simulink model "GradingSystem"  (R2021a)
settings: Solver=FixedStepDiscrete  StartTime=0.0  StopTime=10.0  RelTol=1e-3  EnableMultiTasking=on
settings Model: Creator=Karim  LastModifiedBy=Karim
settings DataIOCC: ReturnWorkspaceOutputs=off
settings OptimizationCC: DefaultParameterBehavior=Inlined  InlineInvariantSignals=on  EnableMemcpy=off  LifeSpan=1  EfficientTunableParamExpr=on
settings DebuggingCC: UnderspecifiedInitializationDetection=Classic  MergeDetectMultiDrivingBlocksExec=none  SFMachineParentedDataDiag=warning  ArithmeticOperatorsInVariantConditions=warning
settings ModelReferenceCC: PropagateSignalLabelsOutOfModel=off
settings SFSimCC: MATLABDynamicMemAlloc=off  CustomCodeUndefinedFunction=UseInterfaceOnly
settings RTWCC: SystemTargetFile=ert.tlc  GenCodeOnly=on  TemplateMakefile=ert_default_tmf  GenerateReport=on  IncludeHyperlinkInReport=on  LaunchReport=on  GenerateTraceInfo=on  GenerateTraceReport=on  GenerateTraceReportSl=on  GenerateTraceReportSf=on  GenerateTraceReportEml=on
settings CodeAppCC: ForceParamTrailComments=on  IgnoreCustomStorageClasses=off  OperatorAnnotations=on  SimulinkDataObjDesc=on  SFDataObjDesc=on  MATLABFcnDesc=on  InsertBlockDesc=on  StateflowObjectComments=on  MATLABSourceComments=on
settings ERTTargetCC: MultiwordLength=2048  GenerateSampleERTMain=on  InlinedParameterPlacement=NonHierarchical  ERTCustomFileTemplate=example_file_process.tlc

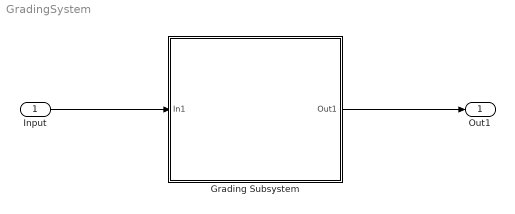
== system GradingSystem ==
  Input : Inport  OutMax=100  OutDataTypeStr=int8
  Grading Subsystem : Subsystem
  Out1 : Outport
  wires:
  Grading Subsystem/1(Out1) -> Out1/1
  Input/1 -> Grading Subsystem/1(In1)

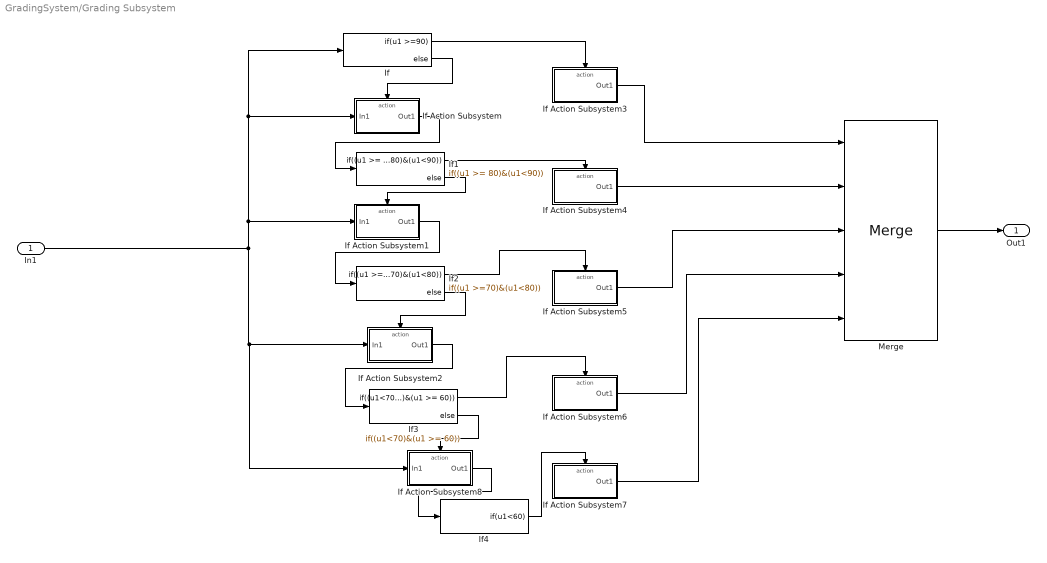
== system GradingSystem/Grading Subsystem ==
  In1 : Inport
  If : If  IfExpression=u1 >=90
  If Action Subsystem : Subsystem  TreatAsAtomicUnit=on
  If Action Subsystem1 : Subsystem  TreatAsAtomicUnit=on
  If Action Subsystem2 : Subsystem  TreatAsAtomicUnit=on
  If Action Subsystem3 : Subsystem  TreatAsAtomicUnit=on
  If Action Subsystem4 : Subsystem  TreatAsAtomicUnit=on
  If Action Subsystem5 : Subsystem  TreatAsAtomicUnit=on
  If Action Subsystem6 : Subsystem  TreatAsAtomicUnit=on
  If Action Subsystem7 : Subsystem  TreatAsAtomicUnit=on
  If Action Subsystem8 : Subsystem  TreatAsAtomicUnit=on
  If1 : If  IfExpression=(u1 >= 80)&(u1<90)
  If2 : If  IfExpression=(u1 >=70)&(u1<80)
  If3 : If  IfExpression=(u1<70)&(u1 >= 60)
  If4 : If  IfExpression=u1<60  ShowElse=off
  Merge : Merge  Inputs=5
  Out1 : Outport
  wires:
  If/2 -> If Action Subsystem/Action
  If Action Subsystem3/1(Out1) -> Merge/1
  If4/1 -> If Action Subsystem7/Action
  If Action Subsystem8/1(Out1) -> If4/1
  If Action Subsystem7/1(Out1) -> Merge/5
  If Action Subsystem5/1(Out1) -> Merge/3
  In1/1 -> If/1, If Action Subsystem/1(In1), If Action Subsystem1/1(In1), If Action Subsystem8/1(In1), If Action Subsystem2/1(In1)
  If Action Subsystem4/1(Out1) -> Merge/2
  If Action Subsystem/1(Out1) -> If1/1
  If Action Subsystem2/1(Out1) -> If3/1
  If Action Subsystem6/1(Out1) -> Merge/4
  If3/2 -> If Action Subsystem8/Action
  If1/2 -> If Action Subsystem1/Action
  If3/1 -> If Action Subsystem6/Action
  If/1 -> If Action Subsystem3/Action
  If2/1 -> If Action Subsystem5/Action
  If Action Subsystem1/1(Out1) -> If2/1
  If2/2 -> If Action Subsystem2/Action
  If1/1 -> If Action Subsystem4/Action
  Merge/1 -> Out1/1

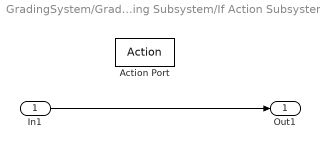
== system GradingSystem/Grading Subsystem/If Action Subsystem ==
  In1 : Inport
  Action Port : ActionPort  ActionPortLabel=else
  Out1 : Outport
  wires:
  In1/1 -> Out1/1

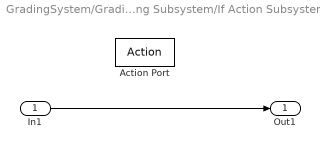
== system GradingSystem/Grading Subsystem/If Action Subsystem1 ==
  In1 : Inport
  Action Port : ActionPort  ActionPortLabel=else
  Out1 : Outport
  wires:
  In1/1 -> Out1/1

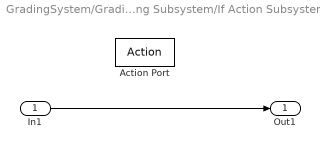
== system GradingSystem/Grading Subsystem/If Action Subsystem2 ==
  In1 : Inport
  Action Port : ActionPort  ActionPortLabel=else
  Out1 : Outport
  wires:
  In1/1 -> Out1/1

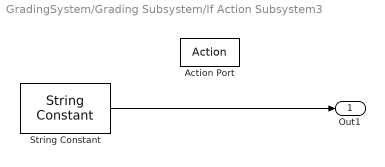
== system GradingSystem/Grading Subsystem/If Action Subsystem3 ==
  Action Port : ActionPort  ActionPortLabel=if(u1 >=90)
  String Constant : StringConstant  String="\"A\""
  Out1 : Outport
  wires:
  String Constant/1 -> Out1/1

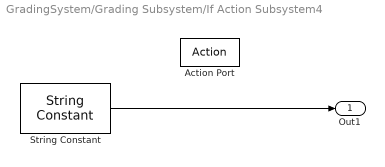
== system GradingSystem/Grading Subsystem/If Action Subsystem4 ==
  Action Port : ActionPort  ActionPortLabel=if((u1 >= 80)&(u1<90))
  String Constant : StringConstant  String="\"B\""
  Out1 : Outport
  wires:
  String Constant/1 -> Out1/1

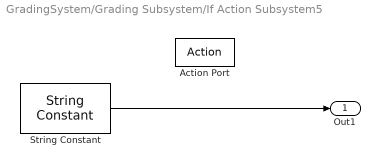
== system GradingSystem/Grading Subsystem/If Action Subsystem5 ==
  Action Port : ActionPort  ActionPortLabel=if((u1 >=70)&(u1<80))
  String Constant : StringConstant  String="\"C\""
  Out1 : Outport
  wires:
  String Constant/1 -> Out1/1

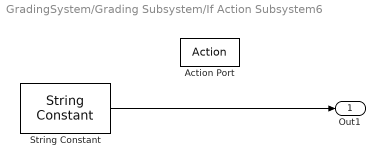
== system GradingSystem/Grading Subsystem/If Action Subsystem6 ==
  Action Port : ActionPort  ActionPortLabel=if((u1<70)&(u1 >= 60))
  String Constant : StringConstant  String="\"D\""
  Out1 : Outport
  wires:
  String Constant/1 -> Out1/1

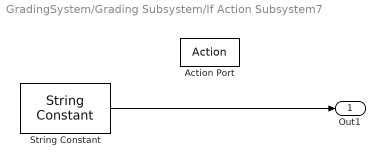
== system GradingSystem/Grading Subsystem/If Action Subsystem7 ==
  Action Port : ActionPort  ActionPortLabel=if(u1<60)
  String Constant : StringConstant  String="\"F\""
  Out1 : Outport
  wires:
  String Constant/1 -> Out1/1

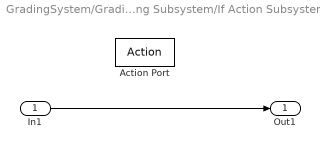
== system GradingSystem/Grading Subsystem/If Action Subsystem8 ==
  In1 : Inport
  Action Port : ActionPort  ActionPortLabel=else
  Out1 : Outport
  wires:
  In1/1 -> Out1/1
